simulink model "Saturazione"  (R2024b)
settings: Solver=VariableStepAuto  StartTime=0.0  StopTime=25  RelTol=1e-3
settings Model: Creator=mcasu  LastModifiedBy=mcasu

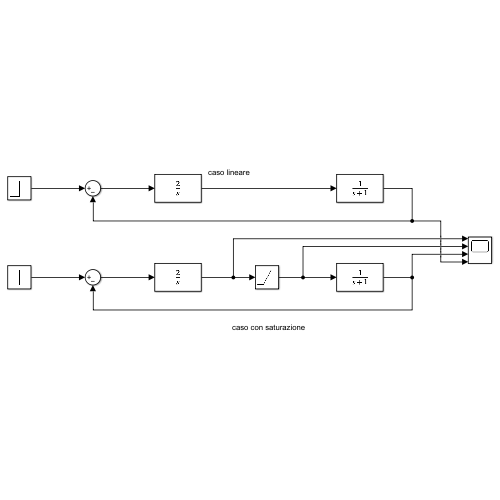
[thumbnail: Simulink's stored preview of the top-level diagram]
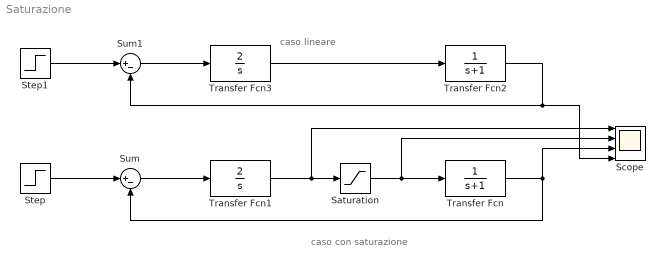
== system Saturazione ==
  note: caso con saturazione
  note: caso lineare
  Saturation : Saturate  UpperLimit=1.05  LowerLimit=-1.05
  Scope : Scope  NumInputPorts=4
  Step : Step  SampleTime=0
  Step1 : Step  SampleTime=0
  Sum : Sum  Inputs=|+-
  Sum1 : Sum  Inputs=|+-
  Transfer Fcn : TransferFcn  Denominator=[1 1]
  Transfer Fcn1 : TransferFcn  Numerator=[2]  Denominator=[1 0]
  Transfer Fcn2 : TransferFcn  Denominator=[1 1]
  Transfer Fcn3 : TransferFcn  Numerator=[2]  Denominator=[1 0]
  wires:
  Transfer Fcn1/1 -> Scope/1, Saturation/1
  Saturation/1 -> Scope/2, Transfer Fcn/1
  Transfer Fcn/1 -> Sum/2, Scope/3
  Sum/1 -> Transfer Fcn1/1
  Step/1 -> Sum/1
  Transfer Fcn2/1 -> Scope/4, Sum1/2
  Sum1/1 -> Transfer Fcn3/1
  Step1/1 -> Sum1/1
  Transfer Fcn3/1 -> Transfer Fcn2/1
